simulink library "hiLvlController_cl"  (R2020a)
settings: Solver=VariableStepAuto  StartTime=0.0  StopTime=10.0  RelTol=1e-3
undefined symbols (not defined in the file): HILVLCONTROLLER, hiLvlCtrl, initializeBussesFromBlock, initializeVariantsFromBlock
libraries: constantBasisParameters_cl x1, calculate_vector_magnitude x1, gpkfPathOpt_cl x1, ilcPathOpt_cl x1, variableAltitudeBasisParams_cl x1, variableRadiusBasisParams_cl x1
settings Model: Creator=mcobb  LastModifiedBy=Ayaz
settings DataIOCC: ReturnWorkspaceOutputs=off
settings DebuggingCC: ArithmeticOperatorsInVariantConditions=warning
settings SFSimCC: CustomCodeUndefinedFunction=UseInterfaceOnly

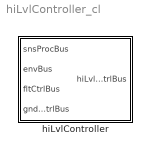
== system hiLvlController_cl ==
  hiLvlController : Subsystem  LoadFcn=initializeVariantsFromBlock(gcb)  InitFcn=initializeVariantsFromBlock(gcb)  StartFcn=initializeVariantsFromBlock(gcb)  Variant=on

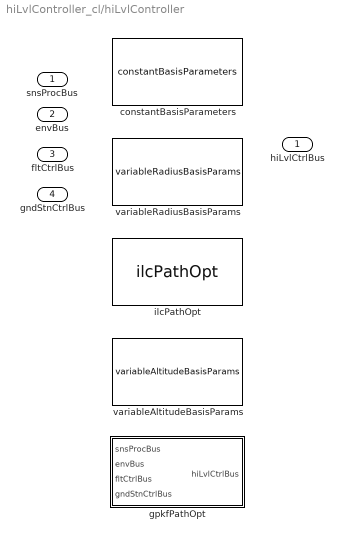
== system hiLvlController_cl/hiLvlController ==
  snsProcBus : Inport  OutDataTypeStr=Bus: sensorsProcessingBus
  envBus : Inport  Port=2  OutDataTypeStr=Bus: envBus
  fltCtrlBus : Inport  Port=3  OutDataTypeStr=Bus: fltCtrlBus
  gndStnCtrlBus : Inport  Port=4  OutDataTypeStr=Bus: gndStnCtrlBus
  constantBasisParameters : constantBasisParameters_cl/constantBasisParameters  VariantControl=strcmpi(HILVLCONTROLLER,'constantBasisParameters')  basisParams=hiLvlCtrl.basisParams.Value
  gpkfPathOpt : Subsystem  LoadFcn=initializeBussesFromBlock(gcb)  InitFcn=initializeBussesFromBlock(gcb)  StartFcn=initializeBussesFromBlock(gcb)  VariantControl=strcmpi(HILVLCONTROLLER,'gpkfPathOpt')  mask{hiLvlCtrl=hiLvlCtrl}
      mask prompts: hiLvlCtrl "Hi-level controller object"
      mask TypeOptions hiLvlCtrl: gpkfPathOpt/hiLvlCtrl
  ilcPathOpt : ilcPathOpt_cl/ilcPathOpt  VariantControl=strcmpi(HILVLCONTROLLER,'ilcPathOpt')  ctrl=hiLvlCtrl
  variableAltitudeBasisParams : variableAltitudeBasisParams_cl/variableAltitudeBasisParams  VariantControl=strcmpi(HILVLCONTROLLER,'variableAltitudeBasisParams')  basisParams=hiLvlCtrl.basisParams.Value
  variableRadiusBasisParams : variableRadiusBasisParams_cl/variableRadiusBasisParams  VariantControl=strcmpi(HILVLCONTROLLER,'variableRadiusBasisParams')  basisParams=hiLvlCtrl.basisParams.Value
  hiLvlCtrlBus : Outport  OutDataTypeStr=Bus: hiLvlCtrlBus  VectorParamsAs1DForOutWhenUnconnected=off

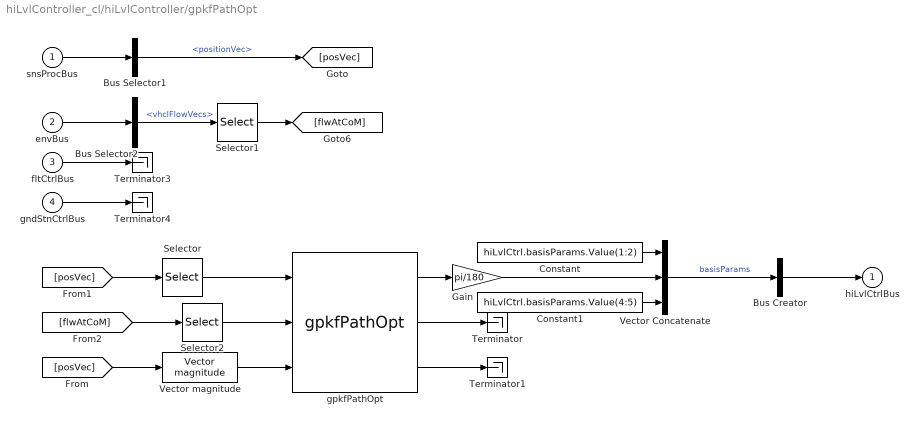
== system hiLvlController_cl/hiLvlController/gpkfPathOpt ==
  snsProcBus : Inport
  envBus : Inport  Port=2
  fltCtrlBus : Inport  Port=3
  gndStnCtrlBus : Inport  Port=4
  Bus Creator : BusCreator  Inputs=1  OutDataTypeStr=Bus: hiLvlCtrlBus
  Bus Selector1 : BusSelector  OutputSignals=positionVec
  Bus Selector2 : BusSelector  OutputSignals=vhclFlowVecs
  Constant : Constant  Value=hiLvlCtrl.basisParams.Value(1:2)
  Constant1 : Constant  Value=hiLvlCtrl.basisParams.Value(4:5)
  Gain : Gain  Gain=pi/180
  Selector : Selector  NumberOfDimensions=2  InputPortWidth=3  IndexOptions=Index vector (dialog),Index vector (dialog)  Indices=3,1  OutputSizes=1,1
  Selector1 : Selector  NumberOfDimensions=2  InputPortWidth=3  IndexOptions=Select all,Index vector (dialog)  Indices=[1 3],5  OutputSizes=1,1
  Selector2 : Selector  NumberOfDimensions=2  InputPortWidth=3  IndexOptions=Index vector (dialog),Index vector (dialog)  Indices=1,1  OutputSizes=1,1
  Terminator{,1,3..4} (4 alike) : Terminator
  Vector Concatenate : Concatenate  NumInputs=3
  Vector magnitude : calculate_vector_magnitude/Vector magnitude  SystemSampleTime=-1  Latency=0  AutoFrameSizeCalculation=off
  gpkfPathOpt : gpkfPathOpt_cl/gpkfPathOpt  hiLvlCtrl=hiLvlCtrl
  hiLvlCtrlBus : Outport
  wires:
  Vector Concatenate/1 -> Bus Creator/1  "basisParams"
  gpkfPathOpt/2 -> Terminator/1
  gpkfPathOpt/3 -> Terminator1/1
  Bus Creator/1 -> hiLvlCtrlBus/1
  snsProcBus/1 -> Bus Selector1/1
  envBus/1 -> Bus Selector2/1
  gndStnCtrlBus/1 -> Terminator4/1
  fltCtrlBus/1 -> Terminator3/1
  Bus Selector1/1 -> [posVec]  "<positionVec>"
  [posVec] -> Vector magnitude/1
  Vector magnitude/1 -> gpkfPathOpt/3
  [posVec] -> Selector/1
  Selector/1 -> gpkfPathOpt/1
  Bus Selector2/1 -> Selector1/1  "<vhclFlowVecs>"
  Selector1/1 -> [flwAtCoM]
  [flwAtCoM] -> Selector2/1
  gpkfPathOpt/1 -> Gain/1
  Constant/1 -> Vector Concatenate/1
  Constant1/1 -> Vector Concatenate/3
  Selector2/1 -> gpkfPathOpt/2
  Gain/1 -> Vector Concatenate/2
